simulink model "EJ3"  (R2021a)
settings: Solver=ode8  StartTime=0.0  StopTime=30  FixedStep=Ts  RelTol=1e-3
values from neighbouring files (symbols this model uses):
  Ts = 20e-3    (= 0.02)    [EJ1_RES.m]    (also in EJ2_RES.m = (4 / wgc) * tan(fase_dig / 2); EJ3_RES.m = (4 / wgc) * tan(fase_dig / 2); EJ4_RES.m = (4 / wgc) * tan(fase_dig / 2))
  ue = wn^3 * x3e    (= -124025106.721)    [EJ2_RES.m]    (also in EJ3_RES.m = 1)
  x1e = pi / 6    (= 0.523598775598)    [EJ2_RES.m]    (also in EJ3_RES.m = 2)
  x2e = 0    [EJ2_RES.m]    (also in EJ3_RES.m = 1)
  ye = x1e    (= 0.523598775598)    [EJ2_RES.m]    (also in EJ3_RES.m = 1)
libraries: cstblocks x1
settings Model: Creator=aghersin  LastModifiedBy=Marce
settings SolverCC: AlgebraicLoopSolver=TrustRegion
settings DataIOCC: ReturnWorkspaceOutputs=off
settings OptimizationCC: LifeSpan=inf
settings DebuggingCC: SFExecutionAtInitializationDiag=none  SFMachineParentedDataDiag=warning  ArithmeticOperatorsInVariantConditions=warning
settings SFSimCC: SimUseLocalCustomCode=off  CustomCodeUndefinedFunction=UseInterfaceOnly
settings RTWCC: RTWUseLocalCustomCode=off
settings CodeAppCC: StateflowObjectComments=on

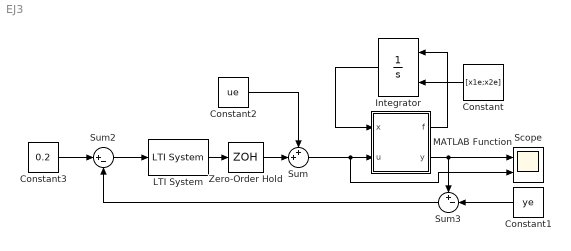
== system EJ3 ==
  Constant : Constant  Value=[x1e;x2e]  VectorParams1D=off
  Constant1 : Constant  Value=ye
  Constant2 : Constant  Value=ue
  Constant3 : Constant  Value=0.2
  Integrator : Integrator  InitialConditionSource=external
  LTI System : cstblocks/LTI System  sys=C_digital  IC=[]
  MATLAB Function : MATLAB Function  TreatAsAtomicUnit=on
  Scope : Scope  NumInputPorts=2
  Sum : Sum  Inputs=++|
  Sum2 : Sum  Inputs=|+-
  Sum3 : Sum  Inputs=+-|
  Zero-Order Hold : ZeroOrderHold  SampleTime=Ts
  wires:
  LTI System/1 -> Zero-Order Hold/1
  Constant2/1 -> Sum/1
  Sum2/1 -> LTI System/1
  MATLAB Function/1(f) -> Integrator/1
  Constant3/1 -> Sum2/1
  Sum3/1 -> Sum2/2
  Constant/1 -> Integrator/2
  MATLAB Function/2(y) -> Sum3/1, Scope/1
  Constant1/1 -> Sum3/2
  Zero-Order Hold/1 -> Sum/2
  Sum/1 -> Scope/2, MATLAB Function/2(u)
  Integrator/1 -> MATLAB Function/1(x)

== matlab function EJ3/MATLAB Function ==
  data: x input; u input; f output; y output
function [f,y] = fcn(x,u)

f1 = -sqrt(abs(x(1) - x(2))) + u;
f2 = sqrt(abs(x(1) - x(2))) - sqrt(x(2));

f=[f1; f2];

y=x(2);
